simulink model "Ball_and_Beam_black_box"  (R2018a)
settings: Solver=VariableStepAuto  StartTime=0.0  StopTime=15  RelTol=1e-3
libraries: slident x2
settings Model: Creator=Zeljko  LastModifiedBy=Zeljko

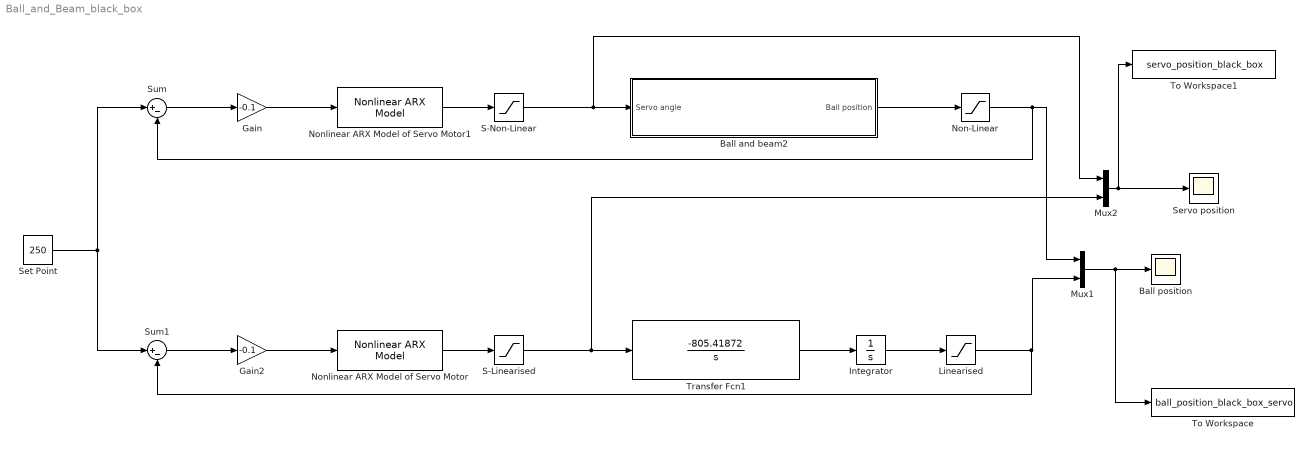
== system Ball_and_Beam_black_box ==
  Ball and beam2 : Subsystem
  Ball position : Scope
  Gain : Gain  Gain=-0.1
  Gain2 : Gain  Gain=-0.1
  Integrator : Integrator  InitialCondition=100
  Linearised : Saturate  UpperLimit=400  LowerLimit=0
  Mux1 : Mux  Inputs=2
  Mux2 : Mux  Inputs=2
  Non-Linear : Saturate  UpperLimit=400  LowerLimit=0
  Nonlinear ARX Model of Servo Motor : slident/Models/Nonlinear ARX Model  sys=sys  ICspec=State values  X0=[0;0;0;0;0;0;0]  U0=0  Y0=0
      settings: SourceProductName=System Identification Toolbox  SourceProductBaseCode=ID
  Nonlinear ARX Model of Servo Motor1 : slident/Models/Nonlinear ARX Model  sys=sys  ICspec=State values  X0=[0;0;0;0;0;0;0]  U0=0  Y0=0
      settings: SourceProductName=System Identification Toolbox  SourceProductBaseCode=ID
  S-Linearised : Saturate  UpperLimit=45  LowerLimit=-45
  S-Non-Linear : Saturate  UpperLimit=45  LowerLimit=-45
  Servo position : Scope
  Set Point : Constant  Value=250
  Sum : Sum  Inputs=|+-
  Sum1 : Sum  Inputs=|+-
  To Workspace : ToWorkspace  VariableName=ball_position_black_box_servo  SaveFormat=Timeseries  SampleTime=-1
  To Workspace1 : ToWorkspace  VariableName=servo_position_black_box  SaveFormat=Timeseries  SampleTime=-1
  Transfer Fcn1 : TransferFcn  Numerator=[-805.41872]  Denominator=[1 0]
  wires:
  Nonlinear ARX Model of Servo Motor1/1 -> S-Non-Linear/1
  S-Non-Linear/1 -> Ball and beam2/1(Servo angle), Mux2/1
  Non-Linear/1 -> Sum/2, Mux1/1
  Sum/1 -> Gain/1
  Gain/1 -> Nonlinear ARX Model of Servo Motor1/1
  Mux1/1 -> Ball position/1, To Workspace/1
  S-Linearised/1 -> Transfer Fcn1/1, Mux2/2
  Sum1/1 -> Gain2/1
  Set Point/1 -> Sum/1, Sum1/1
  Linearised/1 -> Sum1/2, Mux1/2
  Gain2/1 -> Nonlinear ARX Model of Servo Motor/1
  Nonlinear ARX Model of Servo Motor/1 -> S-Linearised/1
  Mux2/1 -> To Workspace1/1, Servo position/1
  Ball and beam2/1(Ball position) -> Non-Linear/1
  Transfer Fcn1/1 -> Integrator/1
  Integrator/1 -> Linearised/1

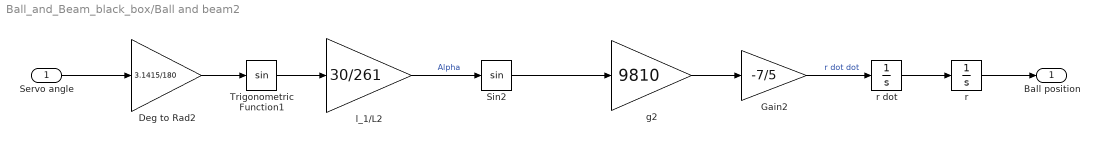
== system Ball_and_Beam_black_box/Ball and beam2 ==
  Servo angle : Inport
  Deg to Rad2 : Gain  Gain=3.1415/180
  Gain2 : Gain  Gain=-7/5
  Sin2 : Trigonometry
  Trigonometric Function1 : Trigonometry
  g2 : Gain  Gain=9810
  l_1/L2 : Gain  Gain=30/261
  r : Integrator  InitialCondition=100
  r dot : Integrator
  Ball position : Outport
  wires:
  Servo angle/1 -> Deg to Rad2/1
  r/1 -> Ball position/1
  Gain2/1 -> r dot/1  "r dot dot"
  Trigonometric Function1/1 -> l_1/L2/1
  l_1/L2/1 -> Sin2/1  "Alpha"
  r dot/1 -> r/1
  Deg to Rad2/1 -> Trigonometric Function1/1
  Sin2/1 -> g2/1
  g2/1 -> Gain2/1
